simulink library "Quintic_Polynomial_Trajectory_Library"  (R2021a)
settings: Solver=VariableStepAuto  StartTime=0.0  StopTime=10.0  RelTol=1e-3
settings Model: Creator=20174215  LastModifiedBy=20174215
settings SolverCC: AlgebraicLoopSolver=TrustRegion
settings DebuggingCC: SFMachineParentedDataDiag=warning

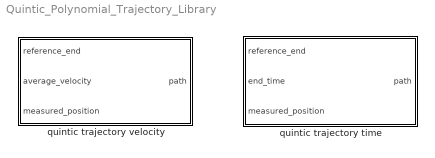
== system Quintic_Polynomial_Trajectory_Library ==
  quintic trajectory time : MATLAB Function  TreatAsAtomicUnit=on
  quintic trajectory velocity : MATLAB Function  TreatAsAtomicUnit=on

== matlab function Quintic_Polynomial_Trajectory_Library/quintic trajectory velocity ==
  data: path output; reference_end input; average_velocity input; Ts parameter; measured_position input
function path = Quintic_Polynomial_Trajectory_Velocity(reference_end, average_velocity, Ts, measured_position)
%% Quintic_Polynomial_Trajectory(reference_end, average_velocity)
% This function outputs a quintic polynomial trajectory over time in 
% Simulink given the end reference and average velocity. The starting 
% velocity and acceleration are set to zero.
%
% Input Arguments
% reference_end = desired end position of the trajectory
% average_velocity = average velocity of the trajectory
% measured_position = current position of the robot arm
%
% Output Arguments
% path = path of the trajectory over time
%
% Quinten Swaan 17-08-2022
%
% Control Systems Technology group
% Departement of Mechanical Engineering
% Eindhoven University of Technology


persistent previous_value_reference_start previous_value_reference_end ...
    path_array index 

if isempty(previous_value_reference_start)
    previous_value_reference_start = 0;
end

if isempty(previous_value_reference_end)
    previous_value_reference_end = 0;
end

if isempty(path_array)
    path_array = zeros(1,1);
end

if isempty(index)
    index = 1;
end


% Obtain new trajectory if a new end reference is given
if previous_value_reference_end ~= reference_end
    t0 = 0;                                 %Starting time
    q0 = previous_value_reference_start;    %Starting position
    v0 = 0;                                 %Starting velocity
    ac0 = 0;                                %Starting acceleration
    tf = abs(previous_value_reference_start-reference_end) / ...
        average_velocity;                   %End time
    qf = reference_end;                     %End position
    vf = 0;                                 %End velocity
    acf = 0;                                %End acceleration

    M = [1 t0 t0^2 t0^3 t0^4 t0^5;
    0 1 2*t0 3*t0^2 4*t0^3 5*t0^4;
    0 0 2 6*t0 12*t0^2 20*t0^3;
    1 tf tf^2 tf^3 tf^4 tf^5;
    0 1 2*tf 3*tf^2 4*tf^3 5*tf^4;
    0 0 2 6*tf 12*tf^2 20*tf^3];

    b = [q0; v0; ac0; qf; vf; acf];

    x = M \ b;

    t = t0:Ts:tf;

    path_array = x(1) + x(2).*t + x(3).*t.^2 + x(4).*t.^3 + +x(5).*t.^4 + x(6).*t.^5;

    index = 1;
    reference_current = path_array(index);

% Output the reference per timestep
else
    if index < length(path_array)
        index = index + 1;
    end
    reference_current = path_array(index);
end

previous_value_reference_end = reference_end;
previous_value_reference_start = measured_position;

path = reference_current;

== matlab function Quintic_Polynomial_Trajectory_Library/quintic trajectory time ==
  data: path output; reference_end input; end_time input; Ts parameter; measured_position input
function path = Quintic_Polynomial_Trajectory_Time(reference_end, end_time, Ts, measured_position)
%% Quintic_Polynomial_Trajectory(reference_end, average_velocity)
% This function outputs a quintic polynomial trajectory over time in 
% Simulink given the end reference and average velocity. The starting 
% velocity and acceleration are set to zero.
%
% Input Arguments
% reference_end = desired end position of the trajectory
% end_time = end time of trajectory; for every new input 
% trajectory starts at time 0 and ends at end_time
% measured_position = current position of the robot arm
%
% Output Arguments
% path = path of the trajectory over time
%
% Quinten Swaan 17-08-2022
%
% Control Systems Technology group
% Departement of Mechanical Engineering
% Eindhoven University of Technology


persistent previous_value_reference_start previous_value_reference_end ...
    path_array index 

if isempty(previous_value_reference_start)
    previous_value_reference_start = 0;
end

if isempty(previous_value_reference_end)
    previous_value_reference_end = 0;
end

if isempty(path_array)
    path_array = zeros(1,1);
end

if isempty(index)
    index = 1;
end


% Obtain new trajectory if a new end reference is given
if previous_value_reference_end ~= reference_end
    t0 = 0;                                 %Starting time
    q0 = previous_value_reference_start;    %Starting position
    v0 = 0;                                 %Starting velocity
    ac0 = 0;                                %Starting acceleration
    tf = end_time;                          %End time
    qf = reference_end;                     %End position
    vf = 0;                                 %End velocity
    acf = 0;                                %End acceleration

    M = [1 t0 t0^2 t0^3 t0^4 t0^5;
    0 1 2*t0 3*t0^2 4*t0^3 5*t0^4;
    0 0 2 6*t0 12*t0^2 20*t0^3;
    1 tf tf^2 tf^3 tf^4 tf^5;
    0 1 2*tf 3*tf^2 4*tf^3 5*tf^4;
    0 0 2 6*tf 12*tf^2 20*tf^3];

    b = [q0; v0; ac0; qf; vf; acf];

    x = M \ b;

    t = t0:Ts:tf;

    path_array = x(1) + x(2).*t + x(3).*t.^2 + x(4).*t.^3 + +x(5).*t.^4 + x(6).*t.^5;

    index = 1;
    reference_current = path_array(index);

% Output the reference per timestep
else
    if index < length(path_array)
        index = index + 1;
    end
    reference_current = path_array(index);
end

previous_value_reference_end = reference_end;
previous_value_reference_start = measured_position;

path = reference_current;
